simulink model "CP_ContrSys_NLin_n9945008"  (R2018b)
settings: Solver=ode4  StartTime=0.0  StopTime=5  FixedStep=0.02  RelTol=1e-3
undefined symbols (not defined in the file): A_NL, B_NL, C_NL, g, K_NL, l, L_NL, m, Mc, x0, xbar
settings Model: Creator=n9945008  LastModifiedBy=n9945008

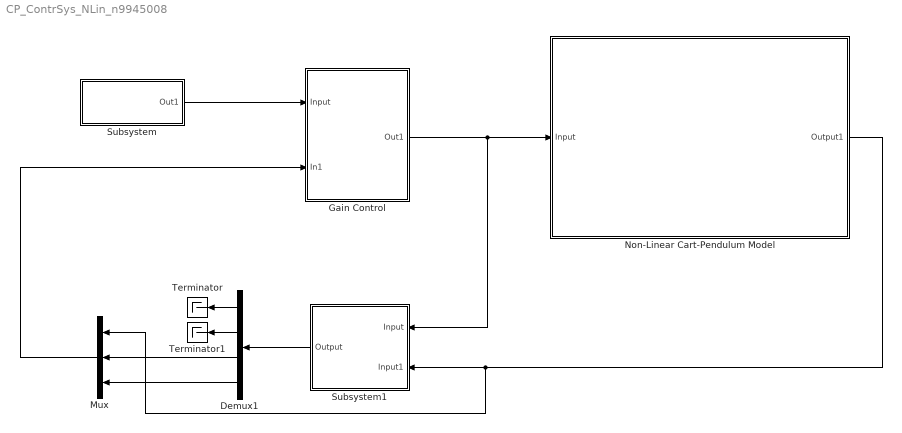
== system CP_ContrSys_NLin_n9945008 ==
  Demux1 : Demux
  Gain Control : Subsystem
  Mux : Mux  Inputs=3
  "Non-Linear Cart-Pendulum Model " : Subsystem
  Subsystem : Subsystem
  Subsystem1 : Subsystem
  Terminator : Terminator
  Terminator1 : Terminator
  wires:
  Subsystem1/1(Output) -> Demux1/1
  Demux1/4 -> Mux/3
  Demux1/1 -> Terminator/1
  Demux1/2 -> Terminator1/1
  Demux1/3 -> Mux/2
  Gain Control/1(Out1) -> Subsystem1/1(Input), "Non-Linear Cart-Pendulum Model "/1(Input)
  Subsystem/1(Out1) -> Gain Control/1(Input)
  Mux/1 -> Gain Control/2(In1)
  "Non-Linear Cart-Pendulum Model "/1(Output1) -> Mux/1, Subsystem1/2(Input1)

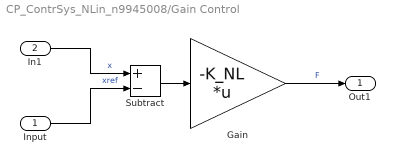
== system CP_ContrSys_NLin_n9945008/Gain Control ==
  Input : Inport
  In1 : Inport  Port=2
  Gain : Gain  Gain=-K_NL  Multiplication=Matrix(K*u)
  Subtract : Sum  Inputs=+-
  Out1 : Outport
  wires:
  Gain/1 -> Out1/1  "F"
  In1/1 -> Subtract/1  "x"
  Input/1 -> Subtract/2  "xref"
  Subtract/1 -> Gain/1

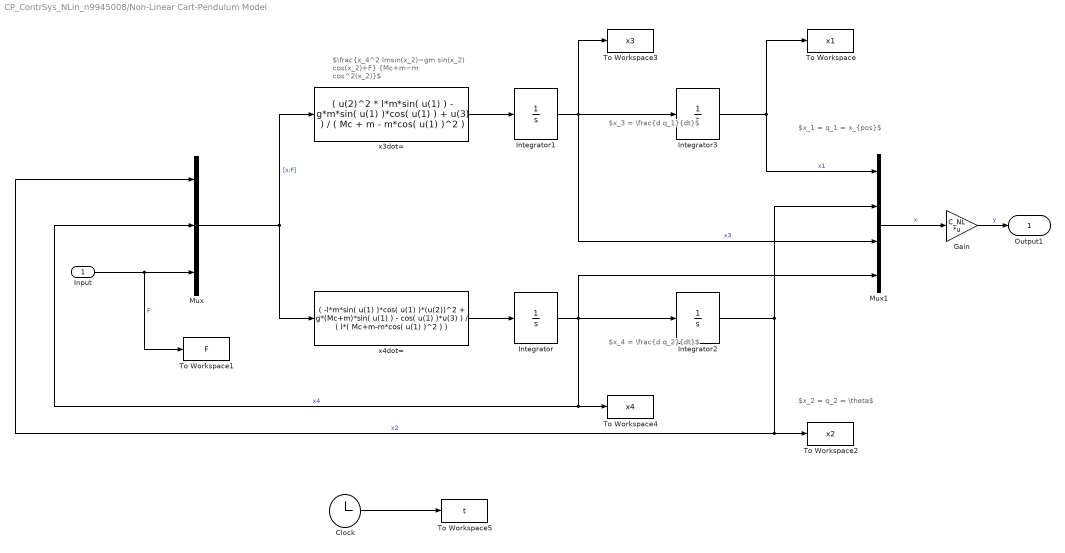
== system CP_ContrSys_NLin_n9945008/Non-Linear Cart-Pendulum Model  ==
  note: $\frac{x_4^2 lmsin(x_2)−gm sin(x_2) cos(x_2)+F} {Mc+m−m cos^2(x_2)}$
  note: $x_4 = \frac{d q_2}{dt}$
  note: $x_3 = \frac{d q_1}{dt}$
  note: $x_1 = q_1 = x_{pos}$
  note: $x_2 = q_2 = \theta$
  Input : Inport
  Clock : Clock
  Gain : Gain  Gain=C_NL  Multiplication=Matrix(K*u)
  Integrator : Integrator  InitialCondition=x0(4)
  Integrator1 : Integrator  InitialCondition=x0(3)
  Integrator2 : Integrator  InitialCondition=x0(2)  WrappedStateUpperValue=2*pi  WrappedStateLowerValue=0
  Integrator3 : Integrator  InitialCondition=x0(1)
  Mux : Mux  Inputs=3
  Mux1 : Mux
  To Workspace : ToWorkspace  VariableName=x1  SampleTime=-1
      settings: Save2DSignal=2-D array (concatenate along first dimension)
  To Workspace1 : ToWorkspace  VariableName=F  SampleTime=-1
      settings: Save2DSignal=2-D array (concatenate along first dimension)
  To Workspace2 : ToWorkspace  VariableName=x2  SampleTime=-1
      settings: Save2DSignal=2-D array (concatenate along first dimension)
  To Workspace3 : ToWorkspace  VariableName=x3  SampleTime=-1
      settings: Save2DSignal=2-D array (concatenate along first dimension)
  To Workspace4 : ToWorkspace  VariableName=x4  SampleTime=-1
      settings: Save2DSignal=2-D array (concatenate along first dimension)
  To Workspace5 : ToWorkspace  VariableName=t  SampleTime=-1
      settings: Save2DSignal=2-D array (concatenate along first dimension)
  "x3dot= " : Fcn  Expr="(  u(2)^2 * l*m*sin( u(1) ) - g*m*sin( u(1) )*cos( u(1) ) + u(3)  )  /  (  Mc + m - m*cos( u(1) )^2  )"
  "x4dot= " : Fcn  Expr="(  -l*m*sin( u(1) )*cos( u(1) )*(u(2))^2 + g*(Mc+m)*sin( u(1) ) - cos( u(1) )*u(3)  )  /  (  l*( Mc+m-m*cos( u(1) )^2 )  )"
  Output1 : Outport
  wires:
  Integrator/1 -> Mux/2, To Workspace4/1, Mux1/4, Integrator2/1  "x4"
  Clock/1 -> To Workspace5/1
  Input/1 -> Mux/3, To Workspace1/1  "F"
  Integrator1/1 -> Mux1/3, Integrator3/1, To Workspace3/1  "x3"
  "x3dot= "/1 -> Integrator1/1
  Mux/1 -> "x4dot= "/1, "x3dot= "/1  "[x;F]"
  "x4dot= "/1 -> Integrator/1
  Integrator3/1 -> Mux1/1, To Workspace/1  "x1"
  Integrator2/1 -> Mux/1, To Workspace2/1, Mux1/2  "x2"
  Mux1/1 -> Gain/1  "x"
  Gain/1 -> Output1/1  "y"

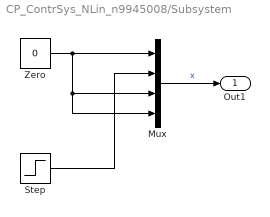
== system CP_ContrSys_NLin_n9945008/Subsystem ==
  Mux : Mux
  Step : Step  Time=0  After=xbar(2)  SampleTime=0
  Zero : Constant  Value=0  OutDataTypeStr=Inherit: Inherit via back propagation
  Out1 : Outport
  wires:
  Mux/1 -> Out1/1  "x"
  Zero/1 -> Mux/4, Mux/3, Mux/1
  Step/1 -> Mux/2

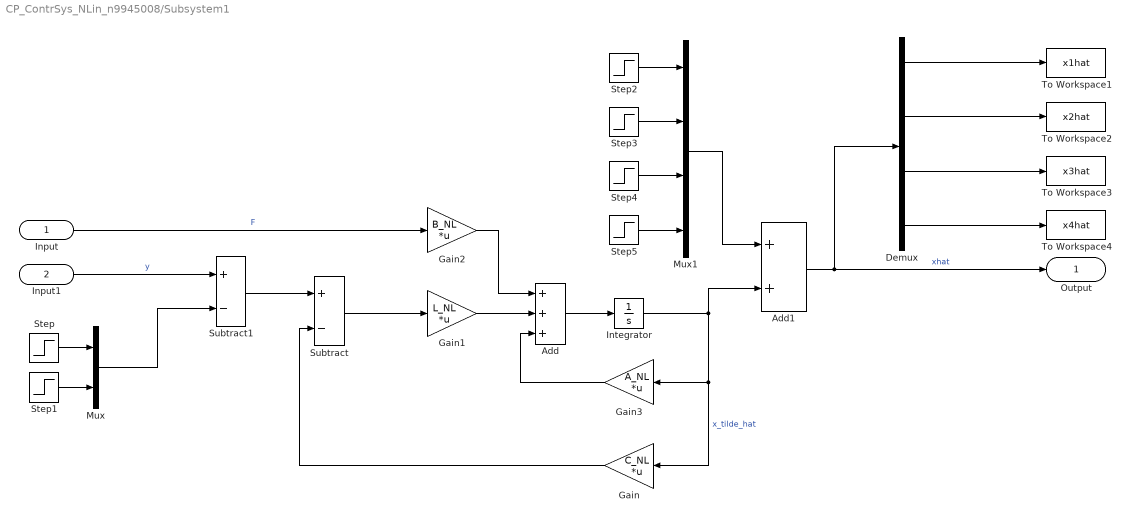
== system CP_ContrSys_NLin_n9945008/Subsystem1 ==
  Input : Inport
  Input1 : Inport  Port=2
  Add : Sum  Inputs=+++
  Add1 : Sum
  Demux : Demux
  Gain : Gain  Gain=C_NL  Multiplication=Matrix(K*u)
  Gain1 : Gain  Gain=L_NL  Multiplication=Matrix(K*u)
  Gain2 : Gain  Gain=B_NL  Multiplication=Matrix(K*u)
  Gain3 : Gain  Gain=A_NL  Multiplication=Matrix(K*u)
  Integrator : Integrator  InitialCondition=x0
  Mux : Mux  Inputs=2
  Mux1 : Mux
  Step : Step  Time=0  After=xbar(1)  SampleTime=0
  Step1 : Step  Time=0  After=xbar(2)  SampleTime=0
  Step2 : Step  Time=0  After=xbar(1)  SampleTime=0
  Step3 : Step  Time=0  After=xbar(2)  SampleTime=0
  Step4 : Step  Time=0  After=xbar(3)  SampleTime=0
  Step5 : Step  Time=0  After=xbar(4)  SampleTime=0
  Subtract : Sum  Inputs=+-
  Subtract1 : Sum  Inputs=+-
  To Workspace1 : ToWorkspace  VariableName=x1hat  SampleTime=-1
      settings: Save2DSignal=2-D array (concatenate along first dimension)
  To Workspace2 : ToWorkspace  VariableName=x2hat  SampleTime=-1
      settings: Save2DSignal=2-D array (concatenate along first dimension)
  To Workspace3 : ToWorkspace  VariableName=x3hat  SampleTime=-1
      settings: Save2DSignal=2-D array (concatenate along first dimension)
  To Workspace4 : ToWorkspace  VariableName=x4hat  SampleTime=-1
      settings: Save2DSignal=2-D array (concatenate along first dimension)
  Output : Outport
  wires:
  Input/1 -> Gain2/1  "F"
  Gain3/1 -> Add/3
  Gain/1 -> Subtract/2
  Gain2/1 -> Add/1
  Demux/4 -> To Workspace4/1
  Demux/2 -> To Workspace2/1
  Subtract/1 -> Gain1/1
  Demux/3 -> To Workspace3/1
  Demux/1 -> To Workspace1/1
  Gain1/1 -> Add/2
  Integrator/1 -> Add1/2, Gain/1, Gain3/1  "x_tilde_hat"
  Add/1 -> Integrator/1
  Input1/1 -> Subtract1/1  "y"
  Subtract1/1 -> Subtract/1
  Step1/1 -> Mux/2
  Step/1 -> Mux/1
  Mux/1 -> Subtract1/2
  Step3/1 -> Mux1/2
  Step2/1 -> Mux1/1
  Step4/1 -> Mux1/3
  Step5/1 -> Mux1/4
  Mux1/1 -> Add1/1
  Add1/1 -> Demux/1, Output/1  "xhat"
